simulink model "sgMdl_IO751_IO752_PROFINETRecord"  (R2024b)
settings: Solver=FixedStepAuto  StartTime=0.0  StopTime=inf  RelTol=1e-3  EnableMultiTasking=on
undefined symbols (not defined in the file): C, Ts_base
libraries: simulink x7, speedgoatlib_IO751 x5, speedgoatlib_IO752 x5
Description:
  | IO751 & IO752 - PROFINET Record
settings Model: ModifiedByFormat=Speedgoat  Creator=Speedgoat  LastModifiedBy=Speedgoat
settings SolverCC: ConcurrentTasks=on  AlgebraicLoopSolver=TrustRegion  PositivePriorityOrder=on  AutoInsertRateTranBlk=on  InsertRTBMode=Never (minimum delay)
settings DataIOCC: SaveFormat=Array  SaveState=on  SignalLoggingName=logsOut
settings OptimizationCC: BlockReduction=off  BooleanDataType=off  OptimizeBlockIOStorage=off  BufferReuse=off  ReuseModelBlockBuffer=off  GlobalBufferReuse=off  ExpressionFolding=off  LocalBlockOutputs=off  InitFltsAndDblsToZero=on  OptimizeDataStoreBuffers=off  BusAssignmentInplaceUpdate=off
settings DebuggingCC: SaveWithParameterizedLinksMsg=none  UnderspecifiedInitializationDetection=Classic  MergeDetectMultiDrivingBlocksExec=none  CheckExecutionContextPreStartOutputMsg=on  SignalResolutionControl=TryResolveAllWithWarning  TasksWithSamePriorityMsg=none  UnconnectedInputMsg=warning  UnconnectedOutputMsg=warning  UnconnectedLineMsg=warning  SFUnexpectedBacktrackingDiag=warning  SFNoUnconditionalDefaultTransitionDiag=warning  SFExecutionAtInitializationDiag=none  ArithmeticOperatorsInVariantConditions=warning
settings HardwareCC: ProdBitPerLong=64  ProdLongLongMode=on  ProdHWDeviceType=Intel->x86-64 (Linux 64)
settings ModelReferenceCC: EnableRefExpFcnMdlSchedulingChecks=on  PropagateSignalLabelsOutOfModel=off
settings SFSimCC: SimUseLocalCustomCode=off  SimTargetLang=C++
settings RTWCC: Description=Speedgoat Real-Time Target Machine  SystemTargetFile=speedgoat.tlc  TemplateMakefile=slrealtime_default_tmf  RTWUseLocalCustomCode=off  Toolchain=Simulink Real-Time Toolchain  BuildConfiguration=Faster Runs  TargetLang=C++  GPUComputeCapability=3.5  DLArmComputeVersion=19.05
settings CodeAppCC: StateflowObjectComments=on
settings SimulinkRealTimeTargetCC: SubcomponentCodeInterfacePackaging=Reusable function  InstructionSetFMA=off  LogToMDFFile=off  SLRTFileLogMaxRuns=10
settings ConfigComp: CovMetricSettings=dw  CovSaveCumulativeToWorkspaceVar=on  CovSaveSingleToWorkspaceVar=on  CovExternalEMLEnable=off  CovSFcnEnable=off  CovBoundaryAbsTol=1.0e-5

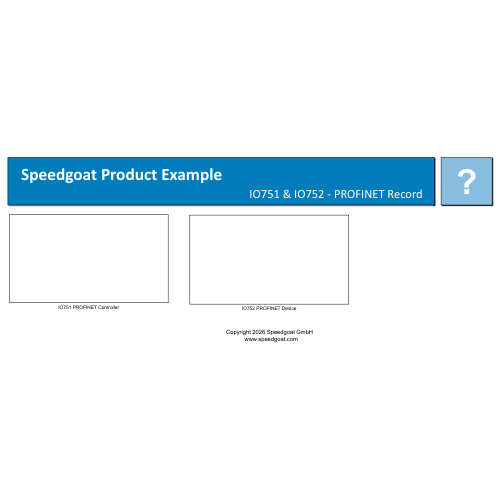
[thumbnail: Simulink's stored preview of the top-level diagram]
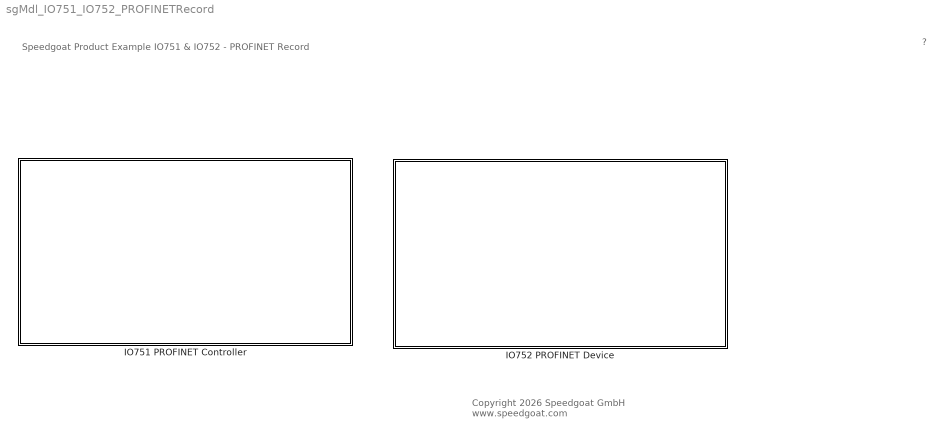
== system sgMdl_IO751_IO752_PROFINETRecord ==
  note: Speedgoat Product Example
      | IO751 & IO752 - PROFINET Record
  note: ?
  note: Copyright 2026 Speedgoat GmbH
      |  www.speedgoat.com
  IO751 PROFINET Controller : Subsystem
  IO752 PROFINET Device : Subsystem

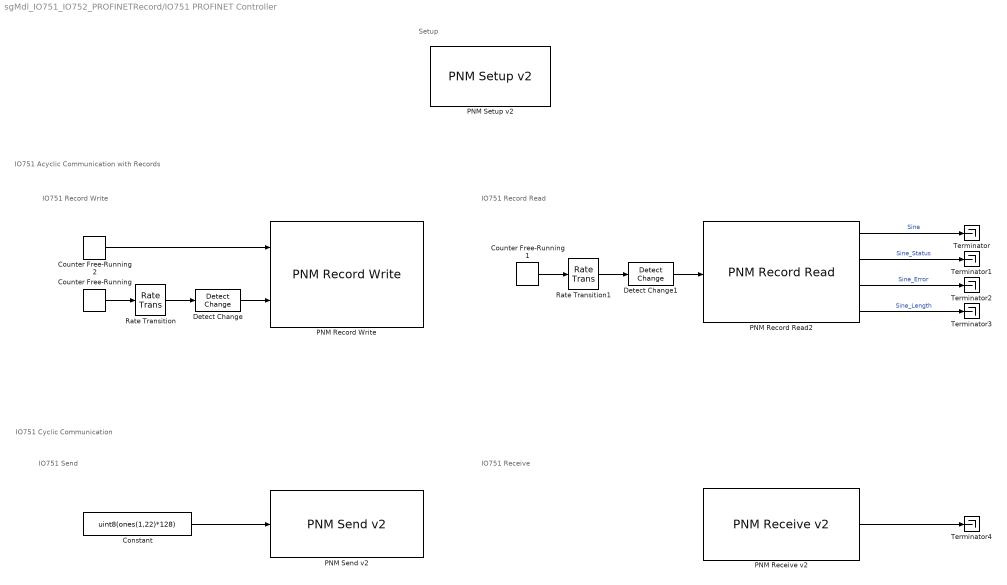
== system sgMdl_IO751_IO752_PROFINETRecord/IO751 PROFINET Controller ==
  note: IO751 Acyclic Communication with Records
  note: Setup
  note: IO751 Record Read
  note: IO751 Record Write
  note: IO751 Send
  note: IO751 Receive
  note: IO751 Cyclic Communication
  Constant : Constant  Value=uint8(ones(1,22)*128)  OutDataTypeStr=Inherit: Inherit via back propagation
  Counter Free-Running : simulink/Sources/Counter Free-Running  NumBits=32  tsamp=Ts_record
  Counter Free-Running1 : simulink/Sources/Counter Free-Running  NumBits=32  tsamp=Ts_record
  Counter Free-Running2 : simulink/Sources/Counter Free-Running  NumBits=32  tsamp=Ts_base
  Detect Change : simulink/Logic and Bit Operations/Detect Change  vinit=0  OutDataTypeStr=boolean
  Detect Change1 : simulink/Logic and Bit Operations/Detect Change  vinit=0  OutDataTypeStr=boolean
  "PNM Receive v2 " : speedgoatlib_IO751/PNM Receive v2   id=1  portType=1 port with n element vector of type UINT8  inputOutput=18  sampleTime=Ts_base
      settings: SourceProductName=IO751 PROFINET Controller
  PNM Record Read2 : speedgoatlib_IO751/PNM Record Read  id=1  DeviceIndex=1  Api=0  Slot=2  SubSlot=1  RecordIndex=3  InitValue=0  parTimeout=100  Extended=on  SampleTime=Ts_base
      settings: SourceProductName=IO751 PROFINET Controller
  PNM Record Write : speedgoatlib_IO751/PNM Record Write  id=1  DeviceIndex=1  Api=0  Slot=1  SubSlot=1  RecordIndex=1  parTimeout=100  Extended=off  SampleTime=Ts_base
      settings: SourceProductName=IO751 PROFINET Controller
  "PNM Send v2 " : speedgoatlib_IO751/PNM Send v2   id=1  portType=1 port with n element vector of type UINT8  inputOutput=22  sampleTime=Ts_base
      settings: SourceProductName=IO751 PROFINET Controller
  "PNM Setup v2 " : speedgoatlib_IO751/PNM Setup v2   id=1  driveLetter=C:  configurationMode=Configuration file  mode=Polling mode  pciSlot=-1  quantityOfAcyclicObjects=0  qtyMods=[1,0,0]  ConfigFile=which('IO751_IO752_Record_m.nxd')  parOptAcyclic=off  protocol=IO751  firmware=PROFINET Controller
      settings: SourceProductName=IO751 PROFINET Controller
  Rate Transition : RateTransition
  Rate Transition1 : RateTransition
  Terminator{,1..4} (5 alike) : Terminator
  wires:
  Detect Change1/1 -> PNM Record Read2/1
  Rate Transition/1 -> Detect Change/1
  Detect Change/1 -> PNM Record Write/2
  Rate Transition1/1 -> Detect Change1/1
  Counter Free-Running2/1 -> PNM Record Write/1
  Counter Free-Running1/1 -> Rate Transition1/1
  Counter Free-Running/1 -> Rate Transition/1
  PNM Record Read2/1 -> Terminator/1  "Sine"
  Constant/1 -> "PNM Send v2 "/1
  "PNM Receive v2 "/1 -> Terminator4/1
  PNM Record Read2/2 -> Terminator1/1  "Sine_Status"
  PNM Record Read2/3 -> Terminator2/1  "Sine_Error"
  PNM Record Read2/4 -> Terminator3/1  "Sine_Length"

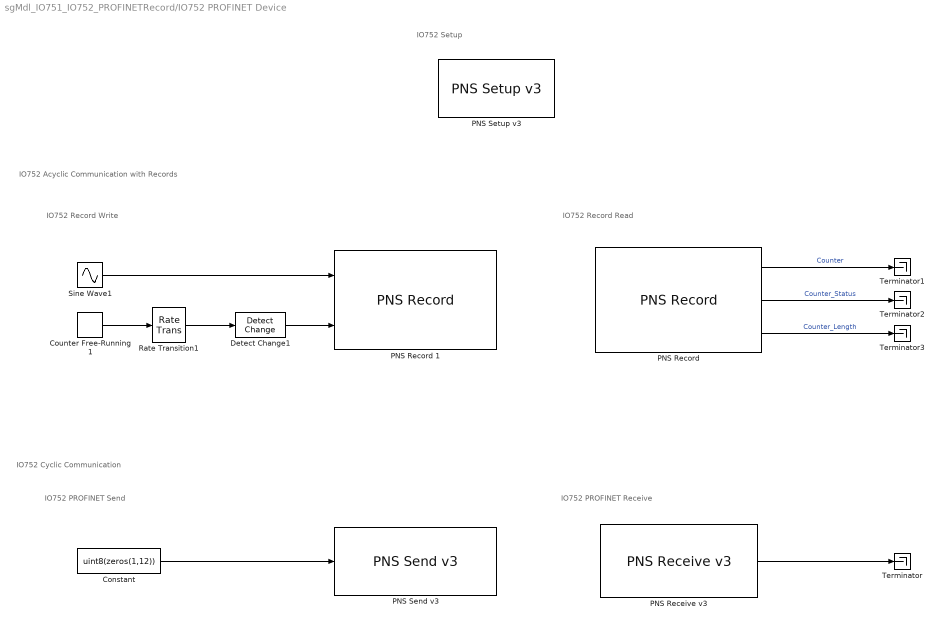
== system sgMdl_IO751_IO752_PROFINETRecord/IO752 PROFINET Device ==
  note: IO752 Setup
  note: IO752 PROFINET Send
  note: IO752 PROFINET Receive
  note: IO752 Acyclic Communication with Records
  note: IO752 Cyclic Communication
  note: IO752 Record Read
  note: IO752 Record Write
  Constant : Constant  Value=uint8(zeros(1,12))
  Counter Free-Running1 : simulink/Sources/Counter Free-Running  NumBits=32  tsamp=Ts_record
  Detect Change1 : simulink/Logic and Bit Operations/Detect Change  vinit=0  OutDataTypeStr=boolean
  PNS Receive v3 : speedgoatlib_IO752/PNS Receive v3  id=2  SampleTime=Ts_base  DataLevel=Device  GroupDataItems=off  PortLabel1=off  PortLabel2=on  PortLabel3=off  PnModuleConfig="{ '0', '', 'CIFX RE/PNS V3.5.35 - V3.x', '8321', '', '', 'DIM 24', '', '', '0', '1', ''; '0', '1', '  CIFX RE/PNS V3.5.35 - V3.x', '8321', '8320', '', 'DIM 24', '1', '', '', '', ''; '0', '32768', '  PN-IO', '8321', '8321', '', 'DIM 24 Interfacesubmodule', '1', '', '', '', ''; '0', '32769', '  Port 1', '8321', '8322', '', 'DIM 24 Portsubmodule 1', '1', '', '', '', ''; '0', '32770', '  Port 2', '8321', '8323', '', 'DIM 24 Portsubmodule 2', '1', '', '', '', ''; '1', '', '12 Bytes Input', '12', '', '', '12byteinput', '0', '', '', '', ''; '1', '1', '  12 Bytes Input', '12', '11', '', '12byteinput', '1', '{\"Inputs\",[3],[12]}', '', '', ''; '2', '', '16 Bytes Output', '15', '', '', '16byteoutput', '0', '', '', '', ''; '2', '1', '  16 Bytes Output', '15', '14', '', '16byteoutput', '1', '', '{\"Outputs\",[3],[16]}', '', '' }"
      settings: SourceProductName=IO752 PROFINET Device
  "PNS Record " : speedgoatlib_IO752/PNS Record   id=2  RecordApi=0  RecordSlot=1  RecordSubSlot=1  RecordIndex=1  RecordInitValue=uint32(0)  ReadOp=on  WriteOp=off  Extended=on  sampleTime=Ts_base
      settings: SourceProductName=IO752 PROFINET Device
  PNS Record 1 : speedgoatlib_IO752/PNS Record   id=2  RecordApi=0  RecordSlot=2  RecordSubSlot=1  RecordIndex=3  RecordInitValue=0  ReadOp=off  WriteOp=on  Extended=off  sampleTime=Ts_base
      settings: SourceProductName=IO752 PROFINET Device
  PNS Send v3 : speedgoatlib_IO752/PNS Send v3  id=2  SampleTime=Ts_base  DataLevel=Device  GroupDataItems=off  PortLabel1=off  PortLabel2=on  PortLabel3=off  PnModuleConfig="{ '0', '', 'CIFX RE/PNS V3.5.35 - V3.x', '8321', '', '', 'DIM 24', '', '', '0', '1', ''; '0', '1', '  CIFX RE/PNS V3.5.35 - V3.x', '8321', '8320', '', 'DIM 24', '1', '', '', '', ''; '0', '32768', '  PN-IO', '8321', '8321', '', 'DIM 24 Interfacesubmodule', '1', '', '', '', ''; '0', '32769', '  Port 1', '8321', '8322', '', 'DIM 24 Portsubmodule 1', '1', '', '', '', ''; '0', '32770', '  Port 2', '8321', '8323', '', 'DIM 24 Portsubmodule 2', '1', '', '', '', ''; '1', '', '12 Bytes Input', '12', '', '', '12byteinput', '0', '', '', '', ''; '1', '1', '  12 Bytes Input', '12', '11', '', '12byteinput', '1', '{\"Inputs\",[3],[12]}', '', '', ''; '2', '', '16 Bytes Output', '15', '', '', '16byteoutput', '0', '', '', '', ''; '2', '1', '  16 Bytes Output', '15', '14', '', '16byteoutput', '1', '', '{\"Outputs\",[3],[16]}', '', '' }"
      settings: SourceProductName=IO752 PROFINET Device
  PNS Setup v3 : speedgoatlib_IO752/PNS Setup v3  id=2  PciSlot=-1  StationName='cifxrepns'  BusStart=On model start  SystemRedundancy=off  RecordSuccess=on  GsdFile=[speedgoatroot, '\sg_blocks\cifx\eds\GSDML-V2.33-HILSCHER-CIFX RE PNS-20170919.xml']  VendorId=286  DeviceId=259  OptionalIdentity=off  DeviceType='cifxrepns'  OrderId='1250.1'  HwRev=2  SwRevPrefix='V'  SwRev=[3,0,0]  SerialNumber='0'  ModuleConfigTable="{ '0', '', 'CIFX RE/PNS V3.5.35 - V3.x', '8321', '', '', 'DIM 24', '', '', '0', '1', ''; '0', '1', '  CIFX RE/PNS V3.5.35 - V3.x', '8321', '8320', '', 'DIM 24', '1', '', '', '', ''; '0', '32768', '  PN-IO', '8321', '8321', '', 'DIM 24 Interfacesubmodule', '1', '', '', '', ''; '0', '32769', '  Port 1', '8321', '8322', '', 'DIM 24 Portsubmodule 1', '1', '', '', '', ''; '0', '32770', '  Port 2', '8321', '8323', '', 'DIM 24 Portsubmodule 2', '1', '', '', '', ''; '1', '', '12 Bytes Input', '12', '', '', '12byteinput', '0', '', '', '', ''; '1', '1', '  12 Bytes Input', '12', '11', '', '12byteinput', '1', '{\"Inputs\",[3],[12]}', '', '', ''; '2', '', '16 Bytes Output', '15', '', '', '16byteoutput', '0', '', '', '', ''; '2', '1', '  16 Bytes Output', '15', '14', '', '16byteoutput', '1', '', '{\"Outputs\",[3],[16]}', '', '' }"
      settings: SourceProductName=IO752 PROFINET Device
  Rate Transition1 : RateTransition
  Sine Wave1 : Sin  SineType=Sample based  Amplitude=10  Frequency=180  Samples=1/0.001*4  SampleTime=Ts_base
  Terminator{,1..3} (4 alike) : Terminator
  wires:
  PNS Receive v3/1 -> Terminator/1
  Constant/1 -> PNS Send v3/1
  "PNS Record "/1 -> Terminator1/1  "Counter"
  "PNS Record "/2 -> Terminator2/1  "Counter_Status"
  "PNS Record "/3 -> Terminator3/1  "Counter_Length"
  Rate Transition1/1 -> Detect Change1/1
  Counter Free-Running1/1 -> Rate Transition1/1
  Detect Change1/1 -> PNS Record 1/2
  Sine Wave1/1 -> PNS Record 1/1
